simulink model "EMT_load"  (R2024a)
settings: Solver=ode1  StartTime=0.0  StopTime=simtime  FixedStep=Ts  RelTol=1e-3
values from neighbouring files (symbols this model uses):
  c0 = c0_hawk    (= 6.37282e-09)    [EMT_Phasor_parameters.m]
  c1 = c1_hawk    (= 8.76156e-09)    [EMT_Phasor_parameters.m]
  fg = 50    [EMT_Phasor_parameters.m]
  G1gen = 0.1245    [EMT_Phasor_parameters.m]
  G2gen = 0.30    (= 0.3)    [EMT_Phasor_parameters.m]
  G3gen = 0.20    (= 0.2)    [EMT_Phasor_parameters.m]
  G4sgen = 0.2078    [EMT_Phasor_parameters.m]
  G5gen = 0.20    (= 0.2)    [EMT_Phasor_parameters.m]
  G6gen = 0.2078    [EMT_Phasor_parameters.m]
  G6sgen = 0.20    (= 0.2)    [EMT_Phasor_parameters.m]
  G7gen = 0.518    [EMT_Phasor_parameters.m]
  Ihvpk = Ihv*sqrt(2)    [EMT_Phasor_parameters.m]
  l0 = l0_hawk    (= 0.00373)    [EMT_Phasor_parameters.m]
  l1 = l1_hawk    (= 0.00133)    [EMT_Phasor_parameters.m]
  L3dem = 0.10    (= 0.1)    [EMT_Phasor_parameters.m]
  L4dem = 0.30    (= 0.3)    [EMT_Phasor_parameters.m]
  L5dem = 0.35    [EMT_Phasor_parameters.m]
  L6dem = 0.15    [EMT_Phasor_parameters.m]
  L7dem = 0.10    (= 0.1)    [EMT_Phasor_parameters.m]
  Pr = Sr*PF    (= 550050000)    [EMT_Phasor_parameters.m]
  Qr = sqrt(Sr^2 - Pr^2)    [EMT_Phasor_parameters.m]
  r0 = r0_hawk    (= 0.44587)    [EMT_Phasor_parameters.m]
  r1 = r1_hawk    (= 0.12087)    [EMT_Phasor_parameters.m]
  Rtpu = Xtpu/40    (= 0.00375)    [EMT_Phasor_parameters.m]
  S1non = 400e6    (= 400000000)    [EMT_Phasor_parameters.m]
  S2non = 300e6    (= 300000000)    [EMT_Phasor_parameters.m]
  S3non = 200e6    (= 200000000)    [EMT_Phasor_parameters.m]
  S4snon = 200e6    (= 200000000)    [EMT_Phasor_parameters.m]
  S5non = 500e6    (= 500000000)    [EMT_Phasor_parameters.m]
  S6non = 400e6    (= 400000000)    [EMT_Phasor_parameters.m]
  S6snon = 200e6    (= 200000000)    [EMT_Phasor_parameters.m]
  S7non = 200e6    (= 200000000)    [EMT_Phasor_parameters.m]
  simtime = 5    [EMT_Phasor_parameters.m]
  tonvsc = 0.01    [EMT_Phasor_parameters.m]
  Ts = 150e-6    (= 0.00015)    [EMT_Phasor_parameters.m]
  Vhv = 220e3    (= 220000)    [EMT_Phasor_parameters.m]
  Vmv = 22e3    (= 22000)    [EMT_Phasor_parameters.m]
  wc1 = wsw1/10    (= 848.230016469)    [EMT_Phasor_parameters.m]
  wdc1 = wc1/10    (= 84.8230016469)    [EMT_Phasor_parameters.m]
  wpq1 = wc1/10    (= 84.8230016469)    [EMT_Phasor_parameters.m]
  wsw1 = ksw1*2*pi*fg    (= 8482.30016469)    [EMT_Phasor_parameters.m]
  Xtpu = 0.15    [EMT_Phasor_parameters.m]
undefined symbols (not defined in the file or in its folder): D11, Delta, Kf, r, theta0
libraries: simulink_extras x152, spsGroundLib x49, spsCurrentMeasurementLib x39, spsVoltageMeasurementLib x33, simulink x32, eeGeneralControl x32, slpidlib x32, powerlib x30, powerlib_meascontrol x28, spsFirstOrderFilterLib x24, eeTransforms x24, pid_lib x16
(part 13 of 16)

== system EMT_load/G5/VSC/VSC Control/Modulation/Phasor I and Phasor PQ/Inverse Park Transform (Phasor) ==
  note: Transforming from real domain to complex domain
  note: In time domain, all variables are real.
      | In phasor domain, they are complex.
      | In phasor domain, what is seen as a variation in real domain is actually an angular displacement
      | As we know that the system is balanced, d and q have the same magnitude and are shifted 90 degrees
      | Thus, having the real parts and knowing that they are shifter 90 degrees, we can recover the complex part
  dq0 : Inport
  theta : Inport  Port=2
  Complex to Magnitude-Angle : ComplexToMagnitudeAngle  Commented=on
  Constant : Constant  Commented=on  Value=exp(-1i*2*pi/3)
  Constant1 : Constant  Commented=on  Value=exp(-1i*4*pi/3)
  Constant2 : Constant  Value=0
  Demux : Demux  Outputs=2
  Demux1 : Demux  Commented=on  Outputs=3
  Exp : Math  OutputSignalType=complex
  Exp1 : Math  Commented=on  OutputSignalType=complex
  First-Order Filter1 : spsFirstOrderFilterLib/First-Order Filter  Commented=on  FilterType=Lowpass  Tc=100e-6  Ts=0  Initialize=off  Vac_Init=[0, 0, 60]  Vdc_Init=0  PlotResponse=off  FreqRange="[0,  200,  1]"
  First-Order Filter2 : spsFirstOrderFilterLib/First-Order Filter  Commented=on  FilterType=Lowpass  Tc=100e-6  Ts=0  Initialize=off  Vac_Init=[0, 0, 60]  Vdc_Init=0  PlotResponse=off  FreqRange="[0,  200,  1]"
  Gain : Gain  Commented=on  Gain=exp(-1i*2*pi/3)
  Gain1 : Gain  Gain=1/2
  Gain2 : Gain  Gain=sqrt(3)
  Gain3 : Gain  Gain=1/2
  Gain4 : Gain  Gain=sqrt(3)
  Gain5 : Gain  Gain=1i
  Gain6 : Gain  Gain=-1
  Gain7 : Gain  Commented=on  Gain=1i
  Gain8 : Gain  Commented=on  Gain=exp(-1i*4*pi/3)
  Magnitude-Angle to Complex : MagnitudeAngleToComplex  Commented=on
  Mux : Mux  Commented=on  Inputs=3
  Mux2 : Mux  Inputs=3
  Product : Product
  Product1 : Product  Commented=on
  Real-Imag to Complex : RealImagToComplex
  Real-Imag to Complex1 : RealImagToComplex
  Sum : Sum  Inputs=|++
  Sum1 : Sum  Inputs=-|-
  Sum2 : Sum  Inputs=-|+
  Terminator : Terminator  Commented=on
  Terminator1 : Terminator  Commented=on
  abc : Outport  VectorParamsAs1DForOutWhenUnconnected=off
  wires:
  ? -> Demux1/1
  Demux1/3 -> Terminator1/1
  Magnitude-Angle to Complex/1 -> Gain/1, Mux/1, Gain8/1
  Gain/1 -> Mux/2
  Complex to Magnitude-Angle/1 -> First-Order Filter1/1
  Demux1/1 -> Complex to Magnitude-Angle/1
  Mux/1 -> ?
  Gain8/1 -> Mux/3
  Demux1/2 -> Terminator/1
  Complex to Magnitude-Angle/2 -> First-Order Filter2/1
  First-Order Filter2/1 -> Magnitude-Angle to Complex/2
  First-Order Filter1/1 -> Magnitude-Angle to Complex/1
  Sum/1 -> abc/1
  Constant2/1 -> [x0]
  Exp1/1 -> Product1/2
  Gain7/1 -> Exp1/1
  Gain6/1 -> Real-Imag to Complex1/2
  [xdr] -> Gain6/1
  [xqr] -> Real-Imag to Complex/2
  [xqr] -> Real-Imag to Complex1/1
  Real-Imag to Complex1/1 -> [xq]
  [xdr] -> Real-Imag to Complex/1
  Real-Imag to Complex/1 -> [xd]
  Gain3/1 -> Mux2/3
  Gain1/1 -> Mux2/2
  Sum2/1 -> Gain3/1
  [xd] -> Gain4/1
  [xq] -> Sum2/1
  Gain4/1 -> Sum2/2
  Gain2/1 -> Sum1/2
  [xd] -> Gain2/1
  [xq] -> Sum1/1
  Sum1/1 -> Gain1/1
  [xq] -> Mux2/1
  theta/1 -> Gain5/1
  Gain5/1 -> Exp/1
  Mux2/1 -> Product/1
  Exp/1 -> Product/2
  Product/1 -> Sum/1
  [x0] -> Sum/2
  Demux/2 -> [xqr]
  Demux/1 -> [xdr]
  dq0/1 -> Demux/1

== system EMT_load/G5/VSC/VSC Control/Modulation/Phasor I and Phasor PQ/RL time constant ==
  note: Adds an RL electrical time constant to the current source
  Id* : Inport
  Iq* : Inport  Port=2
  Cartesian to Polar : simulink_extras/Transformations/Cartesian to Polar
  Corrects delay : Subsystem  Commented=on
  Polar to Cartesian : simulink_extras/Transformations/Polar to Cartesian
  Saturation : Saturate  UpperLimit=Imax  LowerLimit=0
  Sum4 : Sum  Inputs=|++
  Transfer Fcn (with initial outputs) : simulink_extras/Additional Linear/Transfer Fcn (with initial outputs)  Commented=through  N=[1]  D=[L R]  Y0=0  U0=0
  Transfer Fcn (with initial outputs)1 : simulink_extras/Additional Linear/Transfer Fcn (with initial outputs)  Commented=through  N=[1]  D=[L R]  Y0=0  U0=0
  id : Outport  VectorParamsAs1DForOutWhenUnconnected=off
  iq : Outport  Port=2  VectorParamsAs1DForOutWhenUnconnected=off
  wires:
  Corrects delay/1(dphi) -> Sum4/2
  Sum4/1 -> Polar to Cartesian/2
  Cartesian to Polar/2 -> Sum4/1
  Id*/1 -> Transfer Fcn (with initial outputs)/1
  Iq*/1 -> Transfer Fcn (with initial outputs)1/1
  Polar to Cartesian/1 -> id/1
  Polar to Cartesian/2 -> iq/1
  Transfer Fcn (with initial outputs)/1 -> Cartesian to Polar/1
  Transfer Fcn (with initial outputs)1/1 -> Cartesian to Polar/2
  Cartesian to Polar/1 -> Saturation/1
  Saturation/1 -> Polar to Cartesian/1

== system EMT_load/G5/VSC/VSC Control/Modulation/Phasor I and Phasor PQ/Subsystem ==
  note: Symmetrical components to ABC
  012 : Inport
  Gain1 : Gain  Gain=[1 a a2]  SaturateOnIntegerOverflow=on  OutDataTypeStr=Inherit: Same as input  ParamDataTypeStr=Inherit: Same as input
  Gain2 : Gain  Gain=[1 a2 a]  SaturateOnIntegerOverflow=on  OutDataTypeStr=Inherit: Same as input  ParamDataTypeStr=Inherit: Same as input
  Mux : Mux  Inputs=3
  Sum : Sum  Inputs=1  InputSameDT=on  SaturateOnIntegerOverflow=on  OutDataTypeStr=Inherit: Same as first input
  Sum1 : Sum  Inputs=1  InputSameDT=on  SaturateOnIntegerOverflow=on  OutDataTypeStr=Inherit: Same as first input
  Sum2 : Sum  Inputs=1  InputSameDT=on  SaturateOnIntegerOverflow=on  OutDataTypeStr=Inherit: Same as first input
  abc : Outport
  wires:
  Mux/1 -> abc/1
  Sum2/1 -> Mux/1
  Sum/1 -> Mux/2
  Sum1/1 -> Mux/3
  Gain1/1 -> Sum1/1
  012/1 -> Gain2/1, Sum2/1, Gain1/1
  Gain2/1 -> Sum/1

== system EMT_load/G5/VSC/VSC Control/Modulation/Phasor Quasi-EMT/Corrects delay ==
  Clock : Clock
  Gain : Gain  Gain=(2*pi*fg)
  Memory : Memory
  Sum : Sum  Inputs=|+-
  Sum2 : Sum  Inputs=|++
  Transformer connection : Constant  Commented=on  Value=pi/6
  dphi : Outport
  wires:
  Clock/1 -> Memory/1, Sum/1
  Memory/1 -> Sum/2
  Sum/1 -> Gain/1  "Ts"
  Transformer connection/1 -> Sum2/2  "Tf"
  Gain/1 -> Sum2/1
  Sum2/1 -> dphi/1

== system EMT_load/G5/VSC/VSC Control/Modulation/Phasor Quasi-EMT/Corrects delay2 ==
  Clock : Clock
  Gain : Gain  Gain=(2*pi*fg)
  Memory : Memory
  Sum : Sum  Inputs=|+-
  Sum2 : Sum  Inputs=|++
  Transformer connection : Constant  Commented=on  Value=pi/6
  dphi : Outport
  wires:
  Clock/1 -> Memory/1, Sum/1
  Memory/1 -> Sum/2
  Sum/1 -> Gain/1  "Ts"
  Transformer connection/1 -> Sum2/2  "Tf"
  Gain/1 -> Sum2/1
  Sum2/1 -> dphi/1

== system EMT_load/G5/VSC/VSC Control/Modulation/Phasor Quasi-EMT/Inverse Park Transform (Phasor) ==
  note: In time domain, all variables are real.
      | In phasor domain, they are complex.
      | In phasor domain, what is seen as a variation in real domain is actually an angular displacement
      | As we know that the system is balanced, d and q have the same magnitude and are shifted 90 degrees
      | Thus, having the real parts and knowing that they are shifter 90 degrees, we can recover the complex part
  note: Transforming from real domain to complex domain
  dq0 : Inport
  theta : Inport  Port=2
  Complex to Magnitude-Angle : ComplexToMagnitudeAngle  Commented=on
  Constant : Constant  Commented=on  Value=exp(-1i*2*pi/3)
  Constant1 : Constant  Commented=on  Value=exp(-1i*4*pi/3)
  Constant2 : Constant  Value=0
  Demux : Demux  Outputs=2
  Demux1 : Demux  Commented=on  Outputs=3
  Exp : Math  OutputSignalType=complex
  Exp1 : Math  Commented=on  OutputSignalType=complex
  First-Order Filter1 : spsFirstOrderFilterLib/First-Order Filter  Commented=on  FilterType=Lowpass  Tc=100e-6  Ts=0  Initialize=off  Vac_Init=[0, 0, 60]  Vdc_Init=0  PlotResponse=off  FreqRange="[0,  200,  1]"
  First-Order Filter2 : spsFirstOrderFilterLib/First-Order Filter  Commented=on  FilterType=Lowpass  Tc=100e-6  Ts=0  Initialize=off  Vac_Init=[0, 0, 60]  Vdc_Init=0  PlotResponse=off  FreqRange="[0,  200,  1]"
  Gain : Gain  Commented=on  Gain=exp(-1i*2*pi/3)
  Gain1 : Gain  Gain=1/2
  Gain2 : Gain  Gain=sqrt(3)
  Gain3 : Gain  Gain=1/2
  Gain4 : Gain  Gain=sqrt(3)
  Gain5 : Gain  Gain=1i
  Gain6 : Gain  Gain=-1
  Gain7 : Gain  Commented=on  Gain=1i
  Gain8 : Gain  Commented=on  Gain=exp(-1i*4*pi/3)
  Magnitude-Angle to Complex : MagnitudeAngleToComplex  Commented=on
  Mux : Mux  Commented=on  Inputs=3
  Mux2 : Mux  Inputs=3
  Product : Product
  Product1 : Product  Commented=on
  Real-Imag to Complex : RealImagToComplex
  Real-Imag to Complex1 : RealImagToComplex
  Sum : Sum  Inputs=|++
  Sum1 : Sum  Inputs=-|-
  Sum2 : Sum  Inputs=-|+
  Terminator : Terminator  Commented=on
  Terminator1 : Terminator  Commented=on
  abc : Outport  VectorParamsAs1DForOutWhenUnconnected=off
  wires:
  dq0/1 -> Demux/1
  Demux/1 -> [xdr]
  Demux/2 -> [xqr]
  [x0] -> Sum/2
  Product/1 -> Sum/1
  Exp/1 -> Product/2
  Mux2/1 -> Product/1
  Gain5/1 -> Exp/1
  theta/1 -> Gain5/1
  [xq] -> Mux2/1
  Sum1/1 -> Gain1/1
  [xq] -> Sum1/1
  [xd] -> Gain2/1
  Gain2/1 -> Sum1/2
  Gain4/1 -> Sum2/2
  [xq] -> Sum2/1
  [xd] -> Gain4/1
  Sum2/1 -> Gain3/1
  Gain1/1 -> Mux2/2
  Gain3/1 -> Mux2/3
  Real-Imag to Complex/1 -> [xd]
  [xdr] -> Real-Imag to Complex/1
  Real-Imag to Complex1/1 -> [xq]
  [xqr] -> Real-Imag to Complex1/1
  [xqr] -> Real-Imag to Complex/2
  [xdr] -> Gain6/1
  Gain6/1 -> Real-Imag to Complex1/2
  Gain7/1 -> Exp1/1
  Exp1/1 -> Product1/2
  Constant2/1 -> [x0]
  Sum/1 -> abc/1
  First-Order Filter1/1 -> Magnitude-Angle to Complex/1
  First-Order Filter2/1 -> Magnitude-Angle to Complex/2
  Complex to Magnitude-Angle/2 -> First-Order Filter2/1
  Demux1/2 -> Terminator/1
  Gain8/1 -> Mux/3
  Mux/1 -> ?
  Demux1/1 -> Complex to Magnitude-Angle/1
  Complex to Magnitude-Angle/1 -> First-Order Filter1/1
  Gain/1 -> Mux/2
  Magnitude-Angle to Complex/1 -> Gain8/1, Mux/1, Gain/1
  Demux1/3 -> Terminator1/1
  ? -> Demux1/1

== system EMT_load/G5/VSC/VSC Control/Modulation/Phasor Quasi-EMT/Subsystem ==
  note: Symmetrical components to ABC
  012 : Inport
  Gain1 : Gain  Gain=[1 a a2]  SaturateOnIntegerOverflow=on  OutDataTypeStr=Inherit: Same as input  ParamDataTypeStr=Inherit: Same as input
  Gain2 : Gain  Gain=[1 a2 a]  SaturateOnIntegerOverflow=on  OutDataTypeStr=Inherit: Same as input  ParamDataTypeStr=Inherit: Same as input
  Mux : Mux  Inputs=3
  Sum : Sum  Inputs=1  InputSameDT=on  SaturateOnIntegerOverflow=on  OutDataTypeStr=Inherit: Same as first input
  Sum1 : Sum  Inputs=1  InputSameDT=on  SaturateOnIntegerOverflow=on  OutDataTypeStr=Inherit: Same as first input
  Sum2 : Sum  Inputs=1  InputSameDT=on  SaturateOnIntegerOverflow=on  OutDataTypeStr=Inherit: Same as first input
  abc : Outport
  wires:
  Gain2/1 -> Sum/1
  012/1 -> Gain1/1, Sum2/1, Gain2/1
  Gain1/1 -> Sum1/1
  Sum1/1 -> Mux/3
  Sum/1 -> Mux/2
  Sum2/1 -> Mux/1
  Mux/1 -> abc/1

== system EMT_load/G5/VSC/VSC Control/Modulation/Phasor Quasi-EMT/V to I RL (+seq) ==
  note: d-q axis model of a 3-phase series R-L branch
  note: Using Laplace transform:
  note: Iq = (Vq1 - Vq2 - w*L*Id)/(R + s*L)
  note: Id = (Vd1 - Vd2 + w*L*Iq)/(R + s*L)
  note: V2
  note: ==========================================================================================
  note: V1
  note: Vq1 - Vq2 = [ R * Iq ] + [ L* w * Id ] + [ L * d/dt (Iq) ]
  note: where w = 2*pi*f
  note: I --->
  note: o--------| R |---| L |-------o
  note: Vd1 - Vd2 = [ R * Id ] - [ L* w * Iq ] + [ L * d/dt (Id) ]
  note: This subsystem converts the VSC output voltage in a current signal through an RL element
  Vdq1 : Inport
  Vdq2 : Inport  Port=2
  Cartesian to Polar : simulink_extras/Transformations/Cartesian to Polar
  Delay : Delay  DelayLength=1
  Demux : Demux  Outputs=2
  Mux : Mux  Inputs=2
  Polar to Cartesian : simulink_extras/Transformations/Polar to Cartesian
  R_choke1 : Gain  Gain=w*L  SaturateOnIntegerOverflow=on  OutDataTypeStr=Inherit: Same as input  ParamDataTypeStr=Inherit: Same as input
  R_choke2 : Gain  Gain=[1 -1]  SaturateOnIntegerOverflow=on  OutDataTypeStr=Inherit: Same as input  ParamDataTypeStr=Inherit: Same as input
  Saturation : Saturate  UpperLimit=Imax  LowerLimit=0
  Selector : Selector  InputPortWidth=2  IndexOptions=Index vector (dialog)  Indices=[2 1]  OutputSizes=1
  Sum : Sum  Inputs=+-+  SaturateOnIntegerOverflow=on
  Transfer Fcn (with initial outputs) : simulink_extras/Additional Linear/Transfer Fcn (with initial outputs)  N=[1]  D=[L R]  Y0=0  U0=0
  Transfer Fcn (with initial outputs)1 : simulink_extras/Additional Linear/Transfer Fcn (with initial outputs)  N=[1]  D=[L R]  Y0=0  U0=0
  idIq : Outport  VectorParamsAs1DForOutWhenUnconnected=off
  wires:
  Selector/1 -> R_choke1/1
  Vdq1/1 -> Sum/1
  R_choke1/1 -> R_choke2/1
  Sum/1 -> Demux/1
  Demux/1 -> Transfer Fcn (with initial outputs)/1
  Demux/2 -> Transfer Fcn (with initial outputs)1/1
  Polar to Cartesian/1 -> Mux/1
  Polar to Cartesian/2 -> Mux/2
  Cartesian to Polar/2 -> Polar to Cartesian/2
  Mux/1 -> Delay/1, idIq/1
  R_choke2/1 -> Sum/3
  Transfer Fcn (with initial outputs)/1 -> Cartesian to Polar/1
  Transfer Fcn (with initial outputs)1/1 -> Cartesian to Polar/2
  Vdq2/1 -> Sum/2
  Cartesian to Polar/1 -> Saturation/1
  Saturation/1 -> Polar to Cartesian/1
  Delay/1 -> Selector/1

== system EMT_load/G5/VSC/VSC Control/Modulation/Phasor Quasi-EMT/V to I RL (- seq) ==
  note: d-q axis model of a 3-phase series R-L branch
  note: Using Laplace transform:
  note: Iq = (Vq1 - Vq2 - w*L*Id)/(R + s*L)
  note: Id = (Vd1 - Vd2 + w*L*Iq)/(R + s*L)
  note: V2
  note: ==========================================================================================
  note: V1
  note: Vq1 - Vq2 = [ R * Iq ] + [ L* w * Id ] + [ L * d/dt (Iq) ]
  note: where w = 2*pi*f
  note: I --->
  note: o--------| R |---| L |-------o
  note: Vd1 - Vd2 = [ R * Id ] - [ L* w * Iq ] + [ L * d/dt (Id) ]
  note: This subsystem converts the VSC output voltage in a current signal through an RL element
  Vdq1 : Inport
  Vdq2 : Inport  Port=2
  Cartesian to Polar : simulink_extras/Transformations/Cartesian to Polar
  Delay : Delay  DelayLength=1
  Demux : Demux  Outputs=2
  Mux : Mux  Inputs=2
  Polar to Cartesian : simulink_extras/Transformations/Polar to Cartesian
  R_choke1 : Gain  Gain=w*L  SaturateOnIntegerOverflow=on  OutDataTypeStr=Inherit: Same as input  ParamDataTypeStr=Inherit: Same as input
  R_choke2 : Gain  Gain=[-1 1]  SaturateOnIntegerOverflow=on  OutDataTypeStr=Inherit: Same as input  ParamDataTypeStr=Inherit: Same as input
  Saturation : Saturate  UpperLimit=Imax  LowerLimit=0
  Selector : Selector  InputPortWidth=2  IndexOptions=Index vector (dialog)  Indices=[2 1]  OutputSizes=1
  Sum : Sum  Inputs=+-+  SaturateOnIntegerOverflow=on
  Transfer Fcn (with initial outputs) : simulink_extras/Additional Linear/Transfer Fcn (with initial outputs)  N=[1]  D=[L R]  Y0=0  U0=0
  Transfer Fcn (with initial outputs)1 : simulink_extras/Additional Linear/Transfer Fcn (with initial outputs)  N=[1]  D=[L R]  Y0=0  U0=0
  idIq : Outport  VectorParamsAs1DForOutWhenUnconnected=off
  wires:
  Selector/1 -> R_choke1/1
  Vdq1/1 -> Sum/1
  R_choke1/1 -> R_choke2/1
  Sum/1 -> Demux/1
  Demux/1 -> Transfer Fcn (with initial outputs)/1
  Demux/2 -> Transfer Fcn (with initial outputs)1/1
  Polar to Cartesian/1 -> Mux/1
  Polar to Cartesian/2 -> Mux/2
  Cartesian to Polar/2 -> Polar to Cartesian/2
  Mux/1 -> Delay/1, idIq/1
  R_choke2/1 -> Sum/3
  Transfer Fcn (with initial outputs)/1 -> Cartesian to Polar/1
  Transfer Fcn (with initial outputs)1/1 -> Cartesian to Polar/2
  Vdq2/1 -> Sum/2
  Cartesian to Polar/1 -> Saturation/1
  Saturation/1 -> Polar to Cartesian/1
  Delay/1 -> Selector/1

== system EMT_load/G6/VSC/VSC Control/Control loops/Phasor I 1st/Inner-loop ==
  note: Positive-sequence current
  note: Negative-sequence current
  iq+* : Inport
  id+* : Inport  Port=2
  iq-* : Inport  Port=3
  id-* : Inport  Port=4
  First-Order Filter{,1..3} (4 alike) : powerlib_meascontrol/Filters/First-Order Filter  FilterType=Lowpass  Tc=1/wc  Ts=0  Initialize=off  Vac_Init=[0, 0, 60]  Vdc_Init=0  PlotResponse=off  FreqRange="[0,  200,  1]"
  iq+ref : Outport
  id+ref : Outport  Port=2
  iq-ref : Outport  Port=3
  id-ref : Outport  Port=4
  wires:
  First-Order Filter3/1 -> id-ref/1
  id-*/1 -> First-Order Filter3/1
  First-Order Filter2/1 -> iq-ref/1
  iq-*/1 -> First-Order Filter2/1
  First-Order Filter1/1 -> id+ref/1
  id+*/1 -> First-Order Filter1/1
  First-Order Filter/1 -> iq+ref/1
  iq+*/1 -> First-Order Filter/1

== system EMT_load/G6/VSC/VSC Control/Control loops/Phasor I 1st/Outer-loop ==
  note: Limits the converter current
  note: Frequency droop
  note: Voltage droop
  note: Reactive power control
  note: Active power control
  note: LVRT
  Pset : Inport
  Qset : Inport  Port=2
  vqd+- : Inport  Port=3
  iqd+- : Inport  Port=4
  freq : Inport  Port=5
  Blk : Inport  Port=6
  Cartesian to Polar : simulink_extras/Transformations/Cartesian to Polar
  Compare To Constant1 : simulink/Logic and Bit Operations/Compare To Constant  relop=<  const=0  OutDataTypeStr=boolean
  Constant1 : Constant  Value=fg
  Constant10 : Constant  Value=0
  Constant11 : Constant  Value=Vlvrt0
  Constant2 : Constant  Value=Vmvpk
  Constant9 : Constant  Value=0
  Demux : Demux  Outputs=2
  Demux1 : Demux
  Demux2 : Demux
  Gain14 : Gain  Gain=1/Vmvpk
  Gain15 : Gain  Gain=Klvrt
  Gain16 : Gain  Gain=Iconvbase
  Gain5 : Gain  Gain=-1/Kfdroop*(Pconv/fg)
  Gain6 : Gain  Gain=-1/Kvdroop*(Pconv/Vmvpk)
  Mux1 : Mux  Inputs=10
  NOT : Logic  Operator=NOT  IconShape=distinctive  AllPortsSameDT=off  OutDataTypeStr=boolean
  PID Controller1 : pid_lib/PID Controller  Controller=PI  Form=Ideal  TimeDomain=Continuous-time  UseExternalTs=off  SampleTime=-1  IntegratorMethod=Forward Euler  FilterMethod=Forward Euler  ControllerParametersSource=internal  P=kp_pq  I=1/ti_pq  D=0  UseFilter=on  N=100  TunerSelectOption=Transfer Function Based (PID Tuner App)  InitialConditionSource=internal  InitialConditionForIntegrator=0  InitialConditionForFilter=0  DifferentiatorICPrevScaledInput=0  ExternalReset=none  TrackingMode=off  Kt=1  LimitOutput=off  SatLimitsSource=internal  UpperSaturationLimit=inf  LowerSaturationLimit=-inf  LinearizeAsGain=on  AntiWindupMode=none  Kb=1  POutMin=[]  POutMax=[]  IOutMin=[]  IOutMax=[]  DOutMin=[]  DOutMax=[]  NOutMin=[]  NOutMax=[]  SumOutMin=[]  SumOutMax=[]  SaturationOutMin=[]  SaturationOutMax=[]  PParamMin=[]  PParamMax=[]  IParamMin=[]  IParamMax=[]  DParamMin=[]  DParamMax=[]  NParamMin=[]  NParamMax=[]  KbParamMin=[]  KbParamMax=[]  KtParamMin=[]  KtParamMax=[]  KbOutMin=[]  KbOutMax=[]  KtOutMin=[]  KtOutMax=[]  IntegratorOutMin=[]  IntegratorOutMax=[]  FilterOutMin=[]  FilterOutMax=[]  SumI1OutMin=[]  SumI1OutMax=[]  SumI2OutMin=[]  SumI2OutMax=[]  SumI3OutMin=[]  SumI3OutMax=[]  SumI4OutMin=[]  SumI4OutMax=[]  SumDOutMin=[]  SumDOutMax=[]  DifferentiatorOutMin=[]  DifferentiatorOutMax=[]  FilterDiffOutCoefMin=[]  FilterDiffOutCoefMax=[]  ReciprocalOutMin=[]  ReciprocalOutMax=[]  SumDenOutMin=[]  SumDenOutMax=[]  SumNumOutMin=[]  SumNumOutMax=[]  DivideOutMin=[]  DivideOutMax=[]  UdiffTsProdOutMin=[]  UdiffTsProdOutMax=[]  NTsProdOutMin=[]  NTsProdOutMax=[]  UintegralTsProdOutMin=[]  UintegralTsProdOutMax=[]  UngainTsProdOutMin=[]  UngainTsProdOutMax=[]  IntegratorContinuousStateAttributes=''  IntegratorStateMustResolveToSignalObject=off  IntegratorRTWStateStorageClass=Auto  FilterContinuousStateAttributes=''  FilterStateMustResolveToSignalObject=off  FilterRTWStateStorageClass=Auto  ParallelPVariant=Passthrough  IdealPVariant=InternalParameters  IVariant=InternalParameters  DVariant=Disabled  IntegratorVariant=Continuous  SatVariant=Disabled  AWVariant=Passthrough  PCopyVariant=Disabled  TRVariant=Disabled  FdbkBlocksVariant=Forward  IdealPFdbkVariant=Disabled  SatFdbkVariant=Disabled  DerivativeFilterVariant=Disabled  NVariant=Disabled  NCopyVariant=Disabled_SignalSpec  FilterICVariant=Disabled  IntegratorICVariant=InternalICs  ExternalResetVariant=Disabled  TRSumVariant=Passthrough  SumFdbkVariant=Disabled  SumVariant=Sum_PI  TsampFilterVariant=InternalTs  TsampNgainVariant=Passthrough  TsampIntegralVariant=Passthrough  ExternalSaturationOutDataTypeStr=Inherit: Same as second input
  PID Controller6 : pid_lib/PID Controller  Controller=PI  Form=Ideal  TimeDomain=Continuous-time  UseExternalTs=off  SampleTime=-1  IntegratorMethod=Forward Euler  FilterMethod=Forward Euler  ControllerParametersSource=internal  P=kp_pq  I=1/ti_pq  D=0  UseFilter=on  N=100  TunerSelectOption=Transfer Function Based (PID Tuner App)  InitialConditionSource=internal  InitialConditionForIntegrator=0  InitialConditionForFilter=0  DifferentiatorICPrevScaledInput=0  ExternalReset=none  TrackingMode=off  Kt=1  LimitOutput=off  SatLimitsSource=internal  UpperSaturationLimit=inf  LowerSaturationLimit=-inf  LinearizeAsGain=on  AntiWindupMode=none  Kb=1  POutMin=[]  POutMax=[]  IOutMin=[]  IOutMax=[]  DOutMin=[]  DOutMax=[]  NOutMin=[]  NOutMax=[]  SumOutMin=[]  SumOutMax=[]  SaturationOutMin=[]  SaturationOutMax=[]  PParamMin=[]  PParamMax=[]  IParamMin=[]  IParamMax=[]  DParamMin=[]  DParamMax=[]  NParamMin=[]  NParamMax=[]  KbParamMin=[]  KbParamMax=[]  KtParamMin=[]  KtParamMax=[]  KbOutMin=[]  KbOutMax=[]  KtOutMin=[]  KtOutMax=[]  IntegratorOutMin=[]  IntegratorOutMax=[]  FilterOutMin=[]  FilterOutMax=[]  SumI1OutMin=[]  SumI1OutMax=[]  SumI2OutMin=[]  SumI2OutMax=[]  SumI3OutMin=[]  SumI3OutMax=[]  SumI4OutMin=[]  SumI4OutMax=[]  SumDOutMin=[]  SumDOutMax=[]  DifferentiatorOutMin=[]  DifferentiatorOutMax=[]  FilterDiffOutCoefMin=[]  FilterDiffOutCoefMax=[]  ReciprocalOutMin=[]  ReciprocalOutMax=[]  SumDenOutMin=[]  SumDenOutMax=[]  SumNumOutMin=[]  SumNumOutMax=[]  DivideOutMin=[]  DivideOutMax=[]  UdiffTsProdOutMin=[]  UdiffTsProdOutMax=[]  NTsProdOutMin=[]  NTsProdOutMax=[]  UintegralTsProdOutMin=[]  UintegralTsProdOutMax=[]  UngainTsProdOutMin=[]  UngainTsProdOutMax=[]  IntegratorContinuousStateAttributes=''  IntegratorStateMustResolveToSignalObject=off  IntegratorRTWStateStorageClass=Auto  FilterContinuousStateAttributes=''  FilterStateMustResolveToSignalObject=off  FilterRTWStateStorageClass=Auto  ParallelPVariant=Passthrough  IdealPVariant=InternalParameters  IVariant=InternalParameters  DVariant=Disabled  IntegratorVariant=Continuous  SatVariant=Disabled  AWVariant=Passthrough  PCopyVariant=Disabled  TRVariant=Disabled  FdbkBlocksVariant=Forward  IdealPFdbkVariant=Disabled  SatFdbkVariant=Disabled  DerivativeFilterVariant=Disabled  NVariant=Disabled  NCopyVariant=Disabled_SignalSpec  FilterICVariant=Disabled  IntegratorICVariant=InternalICs  ExternalResetVariant=Disabled  TRSumVariant=Passthrough  SumFdbkVariant=Disabled  SumVariant=Sum_PI  TsampFilterVariant=InternalTs  TsampNgainVariant=Passthrough  TsampIntegralVariant=Passthrough  ExternalSaturationOutDataTypeStr=Inherit: Same as second input
  Polar to Cartesian : simulink_extras/Transformations/Polar to Cartesian
  Power calculation : Subsystem
  Product3 : Product
  Saturation : Saturate  UpperLimit=Imax  LowerLimit=0
  Saturation1 : Saturate  UpperLimit=0.1*Pconv  LowerLimit=-0.1*Pconv
  Saturation2 : Saturate  UpperLimit=0.1*Pconv  LowerLimit=-0.1*Pconv
  Saturation7 : Saturate  UpperLimit=0  LowerLimit=-Qmax_lvrt
  Second-Order Filter : eeGeneralControl/Second-Order Filter  FilterType=Low-pass  fn=150  Zeta=0.9  Ts=-1  A0=0  Ph0=0  f0=0  b0=0
  Second-Order Filter1 : eeGeneralControl/Second-Order Filter  FilterType=Low-pass  fn=10  Zeta=0.9  Ts=-1  A0=50  Ph0=0  f0=0.001  b0=50
  Step : Step  Commented=on  Time=0.1  After=0.3*3711  SampleTime=0
  Step1 : Step  Commented=on  Time=0.2  After=0.2*3711  SampleTime=0
  Sum{,4,6,11} (4 alike) : Sum  Inputs=|+-
  Sum2 : Sum  Inputs=-+|
  Sum3 : Sum  Inputs=|++
  Sum5 : Sum  Inputs=|++
  Switch2 : Switch  Threshold=1  SaturateOnIntegerOverflow=off  InputSameDT=off
  Terminator : Terminator
  iq+* : Outport
  id+* : Outport  Port=2
  iq-* : Outport  Port=3
  id-* : Outport  Port=4
  m : Outport  Port=5
  wires:
  Constant10/1 -> id-*/1
  Constant9/1 -> iq-*/1
  Second-Order Filter1/1 -> Sum4/2
  [f] -> Second-Order Filter1/1
  Saturation2/1 -> Sum5/2
  Qset/1 -> Sum5/1
  Cartesian to Polar/2 -> Polar to Cartesian/2
  Polar to Cartesian/1 -> iq+*/1
  Polar to Cartesian/2 -> id+*/1
  Cartesian to Polar/1 -> Saturation/1
  Saturation/1 -> Polar to Cartesian/1
  Demux/1 -> Sum/2  "P"
  Demux/2 -> Sum2/1  "Q"
  Sum3/1 -> Sum/1  "Pref"
  Constant1/1 -> Sum4/1
  Gain5/1 -> Saturation1/1
  Sum4/1 -> Gain5/1
  Saturation1/1 -> Sum3/2
  Sum5/1 -> Sum2/2  "Qref"
  Sum6/1 -> Gain6/1
  Gain6/1 -> Saturation2/1
  [vqfilt] -> Sum6/2
  Constant2/1 -> Sum6/1
  Sum2/1 -> Product3/1
  Pset/1 -> Sum3/1
  PID Controller1/1 -> Cartesian to Polar/1
  Blk/1 -> Terminator/1
  freq/1 -> [f]
  [vqp] -> Mux1/1
  Mux1/1 -> m/1
  Product3/1 -> PID Controller6/1
  Sum/1 -> PID Controller1/1
  Second-Order Filter/1 -> [vqfilt]
  vqd+-/1 -> Demux1/1
  iqd+-/1 -> Demux2/1
  Demux1/1 -> Second-Order Filter/1, [vqp]
  Demux1/2 -> [vdp]
  Demux1/3 -> [vqn]
  Demux1/4 -> [vdn]
  Demux2/1 -> [iqp]
  Demux2/2 -> [idp]
  Demux2/3 -> [iqn]
  Demux2/4 -> [idn]
  [vqp] -> Power calculation/1(vq+)
  [iqp] -> Power calculation/3(iq+)
  Power calculation/1(PQ) -> [PQdq], Demux/1
  [idp] -> Power calculation/4(id+)
  [vdp] -> Power calculation/2(vd+)
  [vqn] -> Power calculation/5(vq-)
  [vdn] -> Power calculation/6(vd-)
  [iqn] -> Power calculation/7(iq-)
  [idn] -> Power calculation/8(id-)
  [LVRT_true] -> NOT/1
  NOT/1 -> Product3/2
  [LVRT_true] -> Switch2/2
  PID Controller6/1 -> Switch2/3
  Switch2/1 -> Cartesian to Polar/2
  Compare To Constant1/1 -> [LVRT_true]
  Gain16/1 -> Switch2/1
  Gain15/1 -> Saturation7/1
  Saturation7/1 -> Compare To Constant1/1, Gain16/1
  [vqfilt] -> Gain14/1
  Sum11/1 -> Gain15/1
  Gain14/1 -> Sum11/2
  Constant11/1 -> Sum11/1
  [vdp] -> Mux1/2
  [vqn] -> Mux1/3
  [vdn] -> Mux1/4
  [iqn] -> Mux1/7
  [idn] -> Mux1/8
  [f] -> Mux1/9
  [PQdq] -> Mux1/10
  [idp] -> Mux1/6
  [iqp] -> Mux1/5

== system EMT_load/G6/VSC/VSC Control/Control loops/Phasor I ref/Outer-loop ==
  note: LVRT
  note: Active power control
  note: Reactive power control
  note: Voltage droop
  note: Frequency droop
  note: Limits the converter current
  Pset : Inport
  Qset : Inport  Port=2
  vqd+- : Inport  Port=3
  iqd+- : Inport  Port=4
  freq : Inport  Port=5
  Blk : Inport  Port=6
  Cartesian to Polar : simulink_extras/Transformations/Cartesian to Polar
  Compare To Constant1 : simulink/Logic and Bit Operations/Compare To Constant  relop=<  const=0  OutDataTypeStr=boolean
  Constant1 : Constant  Value=fg
  Constant10 : Constant  Value=0
  Constant11 : Constant  Value=Vlvrt0
  Constant2 : Constant  Value=Vmvpk
  Constant9 : Constant  Value=0
  Demux : Demux  Outputs=2
  Demux1 : Demux
  Demux2 : Demux
  Gain : Gain  Gain=2/3 * 1/Vmvpk * wpq
  Gain1 : Gain  Gain=2/3 * 1/Vmvpk * wpq
  Gain14 : Gain  Gain=1/Vmvpk
  Gain15 : Gain  Gain=Klvrt
  Gain16 : Gain  Gain=Iconvbase
  Gain5 : Gain  Gain=-1/Kfdroop*(Pconv/fg)
  Gain6 : Gain  Gain=-1/Kvdroop*(Pconv/Vmvpk)
  Integrator : Integrator
  Integrator1 : Integrator
  Mux1 : Mux  Inputs=10
  NOT : Logic  Operator=NOT  IconShape=distinctive  AllPortsSameDT=off  OutDataTypeStr=boolean
  PID Controller1 : pid_lib/PID Controller  Commented=on  Controller=I  Form=Ideal  TimeDomain=Continuous-time  UseExternalTs=off  SampleTime=-1  IntegratorMethod=Forward Euler  FilterMethod=Forward Euler  ControllerParametersSource=internal  P=kp_pq  I=1/wpq  D=0  UseFilter=on  N=100  TunerSelectOption=Transfer Function Based (PID Tuner App)  InitialConditionSource=internal  InitialConditionForIntegrator=0  InitialConditionForFilter=0  DifferentiatorICPrevScaledInput=0  ExternalReset=none  TrackingMode=off  Kt=1  LimitOutput=off  SatLimitsSource=internal  UpperSaturationLimit=inf  LowerSaturationLimit=-inf  LinearizeAsGain=on  AntiWindupMode=none  Kb=1  POutMin=[]  POutMax=[]  IOutMin=[]  IOutMax=[]  DOutMin=[]  DOutMax=[]  NOutMin=[]  NOutMax=[]  SumOutMin=[]  SumOutMax=[]  SaturationOutMin=[]  SaturationOutMax=[]  PParamMin=[]  PParamMax=[]  IParamMin=[]  IParamMax=[]  DParamMin=[]  DParamMax=[]  NParamMin=[]  NParamMax=[]  KbParamMin=[]  KbParamMax=[]  KtParamMin=[]  KtParamMax=[]  KbOutMin=[]  KbOutMax=[]  KtOutMin=[]  KtOutMax=[]  IntegratorOutMin=[]  IntegratorOutMax=[]  FilterOutMin=[]  FilterOutMax=[]  SumI1OutMin=[]  SumI1OutMax=[]  SumI2OutMin=[]  SumI2OutMax=[]  SumI3OutMin=[]  SumI3OutMax=[]  SumI4OutMin=[]  SumI4OutMax=[]  SumDOutMin=[]  SumDOutMax=[]  DifferentiatorOutMin=[]  DifferentiatorOutMax=[]  FilterDiffOutCoefMin=[]  FilterDiffOutCoefMax=[]  ReciprocalOutMin=[]  ReciprocalOutMax=[]  SumDenOutMin=[]  SumDenOutMax=[]  SumNumOutMin=[]  SumNumOutMax=[]  DivideOutMin=[]  DivideOutMax=[]  UdiffTsProdOutMin=[]  UdiffTsProdOutMax=[]  NTsProdOutMin=[]  NTsProdOutMax=[]  UintegralTsProdOutMin=[]  UintegralTsProdOutMax=[]  UngainTsProdOutMin=[]  UngainTsProdOutMax=[]  IntegratorContinuousStateAttributes=''  IntegratorStateMustResolveToSignalObject=off  IntegratorRTWStateStorageClass=Auto  FilterContinuousStateAttributes=''  FilterStateMustResolveToSignalObject=off  FilterRTWStateStorageClass=Auto  ParallelPVariant=Disabled  IdealPVariant=Disabled  IVariant=InternalParameters  DVariant=Disabled  IntegratorVariant=Continuous  SatVariant=Disabled  AWVariant=Passthrough  PCopyVariant=Disabled  TRVariant=Disabled  FdbkBlocksVariant=Forward  IdealPFdbkVariant=Disabled  SatFdbkVariant=Disabled  DerivativeFilterVariant=Disabled  NVariant=Disabled  NCopyVariant=Disabled_SignalSpec  FilterICVariant=Disabled  IntegratorICVariant=InternalICs  ExternalResetVariant=Disabled  TRSumVariant=Passthrough  SumFdbkVariant=Disabled  SumVariant=Passthrough_I  TsampFilterVariant=InternalTs  TsampNgainVariant=Passthrough  TsampIntegralVariant=Passthrough  ExternalSaturationOutDataTypeStr=Inherit: Same as second input
  PID Controller6 : pid_lib/PID Controller  Commented=on  Controller=I  Form=Ideal  TimeDomain=Continuous-time  UseExternalTs=off  SampleTime=-1  IntegratorMethod=Forward Euler  FilterMethod=Forward Euler  ControllerParametersSource=internal  P=kp_pq  I=1/wpq  D=0  UseFilter=on  N=100  TunerSelectOption=Transfer Function Based (PID Tuner App)  InitialConditionSource=internal  InitialConditionForIntegrator=0  InitialConditionForFilter=0  DifferentiatorICPrevScaledInput=0  ExternalReset=none  TrackingMode=off  Kt=1  LimitOutput=off  SatLimitsSource=internal  UpperSaturationLimit=inf  LowerSaturationLimit=-inf  LinearizeAsGain=on  AntiWindupMode=none  Kb=1  POutMin=[]  POutMax=[]  IOutMin=[]  IOutMax=[]  DOutMin=[]  DOutMax=[]  NOutMin=[]  NOutMax=[]  SumOutMin=[]  SumOutMax=[]  SaturationOutMin=[]  SaturationOutMax=[]  PParamMin=[]  PParamMax=[]  IParamMin=[]  IParamMax=[]  DParamMin=[]  DParamMax=[]  NParamMin=[]  NParamMax=[]  KbParamMin=[]  KbParamMax=[]  KtParamMin=[]  KtParamMax=[]  KbOutMin=[]  KbOutMax=[]  KtOutMin=[]  KtOutMax=[]  IntegratorOutMin=[]  IntegratorOutMax=[]  FilterOutMin=[]  FilterOutMax=[]  SumI1OutMin=[]  SumI1OutMax=[]  SumI2OutMin=[]  SumI2OutMax=[]  SumI3OutMin=[]  SumI3OutMax=[]  SumI4OutMin=[]  SumI4OutMax=[]  SumDOutMin=[]  SumDOutMax=[]  DifferentiatorOutMin=[]  DifferentiatorOutMax=[]  FilterDiffOutCoefMin=[]  FilterDiffOutCoefMax=[]  ReciprocalOutMin=[]  ReciprocalOutMax=[]  SumDenOutMin=[]  SumDenOutMax=[]  SumNumOutMin=[]  SumNumOutMax=[]  DivideOutMin=[]  DivideOutMax=[]  UdiffTsProdOutMin=[]  UdiffTsProdOutMax=[]  NTsProdOutMin=[]  NTsProdOutMax=[]  UintegralTsProdOutMin=[]  UintegralTsProdOutMax=[]  UngainTsProdOutMin=[]  UngainTsProdOutMax=[]  IntegratorContinuousStateAttributes=''  IntegratorStateMustResolveToSignalObject=off  IntegratorRTWStateStorageClass=Auto  FilterContinuousStateAttributes=''  FilterStateMustResolveToSignalObject=off  FilterRTWStateStorageClass=Auto  ParallelPVariant=Disabled  IdealPVariant=Disabled  IVariant=InternalParameters  DVariant=Disabled  IntegratorVariant=Continuous  SatVariant=Disabled  AWVariant=Passthrough  PCopyVariant=Disabled  TRVariant=Disabled  FdbkBlocksVariant=Forward  IdealPFdbkVariant=Disabled  SatFdbkVariant=Disabled  DerivativeFilterVariant=Disabled  NVariant=Disabled  NCopyVariant=Disabled_SignalSpec  FilterICVariant=Disabled  IntegratorICVariant=InternalICs  ExternalResetVariant=Disabled  TRSumVariant=Passthrough  SumFdbkVariant=Disabled  SumVariant=Passthrough_I  TsampFilterVariant=InternalTs  TsampNgainVariant=Passthrough  TsampIntegralVariant=Passthrough  ExternalSaturationOutDataTypeStr=Inherit: Same as second input
  Polar to Cartesian : simulink_extras/Transformations/Polar to Cartesian
  Power calculation : Subsystem
  Product3 : Product
  Saturation : Saturate  UpperLimit=Imax  LowerLimit=0
  Saturation1 : Saturate  UpperLimit=0.1*Pconv  LowerLimit=-0.1*Pconv
  Saturation2 : Saturate  UpperLimit=0.1*Pconv  LowerLimit=-0.1*Pconv
  Saturation7 : Saturate  UpperLimit=0  LowerLimit=-Qmax_lvrt
  Second-Order Filter : eeGeneralControl/Second-Order Filter  FilterType=Low-pass  fn=150  Zeta=0.9  Ts=-1  A0=0  Ph0=0  f0=0  b0=0
  Second-Order Filter1 : eeGeneralControl/Second-Order Filter  FilterType=Low-pass  fn=10  Zeta=0.9  Ts=-1  A0=50  Ph0=0  f0=0.001  b0=50
  Step : Step  Commented=on  Time=0.1  After=0.3*3711  SampleTime=0
  Step1 : Step  Commented=on  Time=0.2  After=0.2*3711  SampleTime=0
  Sum{,4,6,11} (4 alike) : Sum  Inputs=|+-
  Sum2 : Sum  Inputs=-+|
  Sum3 : Sum  Inputs=|++
  Sum5 : Sum  Inputs=|++
  Switch2 : Switch  Threshold=1  SaturateOnIntegerOverflow=off  InputSameDT=off
  Terminator : Terminator
  iq+* : Outport
  id+* : Outport  Port=2
  iq-* : Outport  Port=3
  id-* : Outport  Port=4
  m : Outport  Port=5
  wires:
  Gain1/1 -> Integrator1/1
  Gain/1 -> Integrator/1
  NOT/1 -> Product3/2
  [iqp] -> Mux1/5
  [idp] -> Mux1/6
  [PQdq] -> Mux1/10
  [f] -> Mux1/9
  [idn] -> Mux1/8
  [iqn] -> Mux1/7
  [vdn] -> Mux1/4
  [vqn] -> Mux1/3
  [vdp] -> Mux1/2
  Constant11/1 -> Sum11/1
  Gain14/1 -> Sum11/2
  Sum11/1 -> Gain15/1
  [vqfilt] -> Gain14/1
  Saturation7/1 -> Gain16/1, Compare To Constant1/1
  Gain15/1 -> Saturation7/1
  Gain16/1 -> Switch2/1
  Compare To Constant1/1 -> [LVRT_true]
  Switch2/1 -> Cartesian to Polar/2
  Integrator1/1 -> Switch2/3
  [LVRT_true] -> Switch2/2
  [LVRT_true] -> NOT/1
  [idn] -> Power calculation/8(id-)
  [iqn] -> Power calculation/7(iq-)
  [vdn] -> Power calculation/6(vd-)
  [vqn] -> Power calculation/5(vq-)
  [vdp] -> Power calculation/2(vd+)
  [idp] -> Power calculation/4(id+)
  Power calculation/1(PQ) -> Demux/1, [PQdq]
  [iqp] -> Power calculation/3(iq+)
  [vqp] -> Power calculation/1(vq+)
  Demux2/4 -> [idn]
  Demux2/3 -> [iqn]
  Demux2/2 -> [idp]
  Demux2/1 -> [iqp]
  Demux1/4 -> [vdn]
  Demux1/3 -> [vqn]
  Demux1/2 -> [vdp]
  Demux1/1 -> [vqp], Second-Order Filter/1
  iqd+-/1 -> Demux2/1
  vqd+-/1 -> Demux1/1
  Second-Order Filter/1 -> [vqfilt]
  Sum/1 -> Gain/1
  Product3/1 -> Gain1/1
  Mux1/1 -> m/1
  [vqp] -> Mux1/1
  freq/1 -> [f]
  Blk/1 -> Terminator/1
  Integrator/1 -> Cartesian to Polar/1
  Pset/1 -> Sum3/1
  Sum2/1 -> Product3/1
  Constant2/1 -> Sum6/1
  [vqfilt] -> Sum6/2
  Gain6/1 -> Saturation2/1
  Sum6/1 -> Gain6/1
  Sum5/1 -> Sum2/2  "Qref"
  Saturation1/1 -> Sum3/2
  Sum4/1 -> Gain5/1
  Gain5/1 -> Saturation1/1
  Constant1/1 -> Sum4/1
  Sum3/1 -> Sum/1  "Pref"
  Demux/2 -> Sum2/1  "Q"
  Demux/1 -> Sum/2  "P"
  Saturation/1 -> Polar to Cartesian/1
  Cartesian to Polar/1 -> Saturation/1
  Polar to Cartesian/2 -> id+*/1
  Polar to Cartesian/1 -> iq+*/1
  Cartesian to Polar/2 -> Polar to Cartesian/2
  Qset/1 -> Sum5/1
  Saturation2/1 -> Sum5/2
  [f] -> Second-Order Filter1/1
  Second-Order Filter1/1 -> Sum4/2
  Constant9/1 -> iq-*/1
  Constant10/1 -> id-*/1

== system EMT_load/G6/VSC/VSC Control/Control loops/Phasor PQ 1st/Outer-loop ==
  note: Limits the converter current
  note: Frequency droop
  note: Voltage droop
  note: Reactive power control
  note: Active power control
  note: LVRT
  Pset : Inport
  Qset : Inport  Port=2
  vqd+- : Inport  Port=3
  iqd+- : Inport  Port=4
  freq : Inport  Port=5
  Blk : Inport  Port=6
  Cartesian to Polar : simulink_extras/Transformations/Cartesian to Polar
  Compare To Constant1 : simulink/Logic and Bit Operations/Compare To Constant  relop=<  const=0  OutDataTypeStr=boolean
  Constant1 : Constant  Value=fg
  Constant10 : Constant  Value=0
  Constant11 : Constant  Value=Vlvrt0
  Constant2 : Constant  Value=Vmvpk
  Constant9 : Constant  Value=0
  Demux1 : Demux
  Demux2 : Demux
  Divide1 : Product  Inputs=*/
  Divide2 : Product  Inputs=*/
  First-Order Filter : powerlib_meascontrol/Filters/First-Order Filter  FilterType=Lowpass  Tc=1/wpq  Ts=0  Initialize=off  Vac_Init=[0, 0, 60]  Vdc_Init=0  PlotResponse=off  FreqRange="[0,  200,  1]"
  First-Order Filter2 : powerlib_meascontrol/Filters/First-Order Filter  FilterType=Lowpass  Tc=1/wpq  Ts=0  Initialize=off  Vac_Init=[0, 0, 60]  Vdc_Init=0  PlotResponse=off  FreqRange="[0,  200,  1]"
  Gain : Gain  Gain=2/3
  Gain1 : Gain  Gain=2/3
  Gain14 : Gain  Gain=1/Vmvpk
  Gain15 : Gain  Gain=Klvrt
  Gain16 : Gain  Gain=Iconvbase
  Gain5 : Gain  Gain=-1/Kfdroop*(Pconv/fg)
  Gain6 : Gain  Gain=-1/Kvdroop*(Pconv/Vmvpk)
  Mux1 : Mux  Inputs=10
  Polar to Cartesian : simulink_extras/Transformations/Polar to Cartesian
  Power calculation : Subsystem
  Saturation : Saturate  UpperLimit=Imax  LowerLimit=0
  Saturation1 : Saturate  UpperLimit=0.1*Pconv  LowerLimit=-0.1*Pconv
  Saturation2 : Saturate  UpperLimit=0.1*Pconv  LowerLimit=-0.1*Pconv
  Saturation3 : Saturate  UpperLimit=inf  LowerLimit=eps
  Saturation4 : Saturate  UpperLimit=inf  LowerLimit=eps
  Saturation7 : Saturate  UpperLimit=0  LowerLimit=-Qmax_lvrt
  Second-Order Filter : eeGeneralControl/Second-Order Filter  FilterType=Low-pass  fn=150  Zeta=0.9  Ts=-1  A0=0  Ph0=0  f0=0  b0=0
  Second-Order Filter1 : eeGeneralControl/Second-Order Filter  FilterType=Low-pass  fn=10  Zeta=0.9  Ts=-1  A0=50  Ph0=0  f0=0.001  b0=50
  Step : Step  Commented=on  Time=0.1  After=0.3*3711  SampleTime=0
  Step1 : Step  Commented=on  Time=0.2  After=0.2*3711  SampleTime=0
  Sum11 : Sum  Inputs=|+-
  Sum3 : Sum  Inputs=|++
  Sum4 : Sum  Inputs=|+-
  Sum5 : Sum  Inputs=|++
  Sum6 : Sum  Inputs=|+-
  Switch2 : Switch  Threshold=1  SaturateOnIntegerOverflow=off  InputSameDT=off
  Terminator : Terminator
  iq+* : Outport
  id+* : Outport  Port=2
  iq-* : Outport  Port=3
  id-* : Outport  Port=4
  m : Outport  Port=5
  wires:
  [vqp] -> Saturation4/1
  Saturation4/1 -> Divide2/2
  Divide2/1 -> Gain1/1
  Gain1/1 -> First-Order Filter2/1
  Gain/1 -> First-Order Filter/1
  [vqp] -> Saturation3/1
  Divide1/1 -> Gain/1
  Saturation3/1 -> Divide1/2
  Constant10/1 -> id-*/1
  Constant9/1 -> iq-*/1
  Second-Order Filter1/1 -> Sum4/2
  [f] -> Second-Order Filter1/1
  Saturation2/1 -> Sum5/2
  Qset/1 -> Sum5/1
  Cartesian to Polar/2 -> Polar to Cartesian/2
  Polar to Cartesian/1 -> iq+*/1
  Polar to Cartesian/2 -> id+*/1
  Cartesian to Polar/1 -> Saturation/1
  Saturation/1 -> Polar to Cartesian/1
  Sum3/1 -> Divide1/1  "Pref"
  Constant1/1 -> Sum4/1
  Gain5/1 -> Saturation1/1
  Sum4/1 -> Gain5/1
  Saturation1/1 -> Sum3/2
  Sum5/1 -> Divide2/1  "Qref"
  Sum6/1 -> Gain6/1
  Gain6/1 -> Saturation2/1
  [vqfilt] -> Sum6/2
  Constant2/1 -> Sum6/1
  Pset/1 -> Sum3/1
  First-Order Filter/1 -> Cartesian to Polar/1
  Blk/1 -> Terminator/1
  freq/1 -> [f]
  [vqp] -> Mux1/1
  Mux1/1 -> m/1
  Second-Order Filter/1 -> [vqfilt]
  vqd+-/1 -> Demux1/1
  iqd+-/1 -> Demux2/1
  Demux1/1 -> Second-Order Filter/1, [vqp]
  Demux1/2 -> [vdp]
  Demux1/3 -> [vqn]
  Demux1/4 -> [vdn]
  Demux2/1 -> [iqp]
  Demux2/2 -> [idp]
  Demux2/3 -> [iqn]
  Demux2/4 -> [idn]
  [vqp] -> Power calculation/1(vq+)
  [iqp] -> Power calculation/3(iq+)
  Power calculation/1(PQ) -> [PQdq]
  [idp] -> Power calculation/4(id+)
  [vdp] -> Power calculation/2(vd+)
  [vqn] -> Power calculation/5(vq-)
  [vdn] -> Power calculation/6(vd-)
  [iqn] -> Power calculation/7(iq-)
  [idn] -> Power calculation/8(id-)
  [LVRT_true] -> Switch2/2
  First-Order Filter2/1 -> Switch2/3
  Switch2/1 -> Cartesian to Polar/2
  Compare To Constant1/1 -> [LVRT_true]
  Gain16/1 -> Switch2/1
  Gain15/1 -> Saturation7/1
  Saturation7/1 -> Compare To Constant1/1, Gain16/1
  [vqfilt] -> Gain14/1
  Sum11/1 -> Gain15/1
  Gain14/1 -> Sum11/2
  Constant11/1 -> Sum11/1
  [vdp] -> Mux1/2
  [vqn] -> Mux1/3
  [vdn] -> Mux1/4
  [iqn] -> Mux1/7
  [idn] -> Mux1/8
  [f] -> Mux1/9
  [PQdq] -> Mux1/10
  [idp] -> Mux1/6
  [iqp] -> Mux1/5

== system EMT_load/G6/VSC/VSC Control/Control loops/SW, EMT AVG, Phasor Quasi-EMT/Inner-loop ==
  note: Positive-sequence current control
  note: Negative-sequence current control
  iq+* : Inport
  id+* : Inport  Port=2
  iq-* : Inport  Port=3
  id-* : Inport  Port=4
  Blk : Inport  Port=5
  vqd+- : Inport  Port=6
  iqd+- : Inport  Port=7
  Demux1 : Demux
  Demux2 : Demux
  Gain{,1..3} (4 alike) : Gain  Gain=Xt
  NOT{,1..3} (4 alike) : Logic  Operator=NOT  IconShape=distinctive  AllPortsSameDT=off  OutDataTypeStr=boolean
  PID Controller{1..4} (4 alike) : slpidlib/PID Controller  Controller=PI  Form=Ideal  TimeDomain=Continuous-time  UseExternalTs=off  SampleTime=-1  IntegratorMethod=Forward Euler  FilterMethod=Forward Euler  ControllerParametersSource=internal  P=kp_c  I=1/ti_c  UseKiTs=off  D=0  UseExternalDerivativeSource=off  N=100  UseFilter=on  TunerSelectOption=Transfer Function Based (PID Tuner App)  InitialConditionSource=internal  InitialConditionForIntegrator=0  InitialConditionForFilter=0  DifferentiatorICPrevScaledInput=0  ExternalReset=level  TrackingMode=off  Kt=1  LimitOutput=off  SatLimitsSource=internal  UpperSaturationLimit=10*Vmvpk  LowerSaturationLimit=-10*Vmvpk  LinearizeAsGain=off  AntiWindupMode=none  Kb=1  LimitIntegrator=off  UpperIntegratorSaturationLimit=inf  LowerIntegratorSaturationLimit=-inf  POutMin=[]  POutMax=[]  IOutMin=[]  IOutMax=[]  DOutMin=[]  DOutMax=[]  NOutMin=[]  NOutMax=[]  SumOutMin=[]  SumOutMax=[]  SaturationOutMin=[]  SaturationOutMax=[]  PParamMin=[]  PParamMax=[]  IParamMin=[]  IParamMax=[]  DParamMin=[]  DParamMax=[]  NParamMin=[]  NParamMax=[]  KbParamMin=[]  KbParamMax=[]  KtParamMin=[]  KtParamMax=[]  KbOutMin=[]  KbOutMax=[]  KtOutMin=[]  KtOutMax=[]  IntegratorOutMin=[]  IntegratorOutMax=[]  FilterOutMin=[]  FilterOutMax=[]  SumI1OutMin=[]  SumI1OutMax=[]  SumI2OutMin=[]  SumI2OutMax=[]  SumI3OutMin=[]  SumI3OutMax=[]  SumI4OutMin=[]  SumI4OutMax=[]  SumDOutMin=[]  SumDOutMax=[]  DifferentiatorOutMin=[]  DifferentiatorOutMax=[]  FilterDiffOutCoefMin=[]  FilterDiffOutCoefMax=[]  ReciprocalOutMin=[]  ReciprocalOutMax=[]  SumDenOutMin=[]  SumDenOutMax=[]  SumNumOutMin=[]  SumNumOutMax=[]  DivideOutMin=[]  DivideOutMax=[]  UdiffTsProdOutMin=[]  UdiffTsProdOutMax=[]  NTsProdOutMin=[]  NTsProdOutMax=[]  UintegralTsProdOutMin=[]  UintegralTsProdOutMax=[]  UngainTsProdOutMin=[]  UngainTsProdOutMax=[]  ClampingZeroOutDataTypeStr=Inherit: Inherit via back propagation  ClampingZeroOutMin=[]  ClampingZeroOutMax=[]  FilterDenConstantOutDataTypeStr=Inherit: Inherit via back propagation  FilterDenConstantOutMin=[]  FilterDenConstantOutMax=[]  PCopyOutDataTypeStr=Inherit: Inherit via back propagation  PCopyOutMin=[]  PCopyOutMax=[]  NCopyOutDataTypeStr=Inherit: Inherit via back propagation  NCopyOutMin=[]  NCopyOutMax=[]  IntegratorContinuousStateAttributes=''  IntegratorStateMustResolveToSignalObject=off  IntegratorRTWStateStorageClass=Auto  FilterContinuousStateAttributes=''  FilterStateMustResolveToSignalObject=off  FilterRTWStateStorageClass=Auto  ParallelPVariant=Passthrough  IdealPVariant=InternalParameters  IVariant=InternalParameters  DVariant=Disabled  IntegratorVariant=Continuous  SatVariant=Disabled  AWVariant=Passthrough  PCopyVariant=Disabled  TRVariant=Disabled  FdbkBlocksVariant=Forward  IdealPFdbkVariant=Disabled  SatFdbkVariant=Disabled  DerivativeFilterVariant=Disabled  NVariant=Disabled  NCopyVariant=Disabled_SignalSpec  FilterICVariant=Disabled  IntegratorICVariant=InternalICs  ExternalResetVariant=ExternalReset  TRSumVariant=Passthrough  SumFdbkVariant=Disabled  SumVariant=Sum_PI  TsampFilterVariant=InternalTs  TsampNgainVariant=Passthrough  TsampIntegralVariant=Disabled_SignalSpec  ExternalSaturationOutDataTypeStr=Inherit: Same as second input  DerivativeSourceVariant=Disabled
  Product{,1..3} (4 alike) : Product
  Sum : Sum  Inputs=|+-
  Sum1 : Sum  Inputs=+-+
  Sum2 : Sum  Inputs=+--
  Sum3 : Sum  Inputs=-+|
  Sum4 : Sum  Inputs=|+-
  Sum5 : Sum  Inputs=--+
  Sum6 : Sum  Inputs=+-+
  Sum7 : Sum  Inputs=-+|
  vq+* : Outport
  vd+* : Outport  Port=2
  vq-* : Outport  Port=3
  vd-* : Outport  Port=4
  wires:
  [vdp] -> Sum1/3
  iq+*/1 -> Sum/1
  [iqp] -> Gain1/1, Sum/2
  [idp] -> Gain/1, Sum3/1
  PID Controller3/1 -> Sum1/2
  Gain1/1 -> Sum1/1
  PID Controller2/1 -> Sum2/2
  Gain/1 -> Sum2/3
  id+*/1 -> Sum3/2
  Blk/1 -> [blk]
  [blk] -> NOT/1, PID Controller2/2
  Product/1 -> PID Controller2/1
  Sum/1 -> Product/1
  NOT/1 -> Product/2
  [blk] -> PID Controller3/2, NOT1/1
  NOT1/1 -> Product1/2
  Sum3/1 -> Product1/1
  Product1/1 -> PID Controller3/1
  Sum1/1 -> vd+*/1
  Sum2/1 -> vq+*/1
  [vqp] -> Sum2/1
  Demux2/2 -> [idp]
  iqd+-/1 -> Demux2/1
  Demux2/4 -> [idn]
  Demux1/3 -> [vqn]
  Demux1/2 -> [vdp]
  Demux1/4 -> [vdn]
  Demux1/1 -> [vqp]
  Demux2/3 -> [iqn]
  Demux2/1 -> [iqp]
  vqd+-/1 -> Demux1/1
  iq-*/1 -> Sum4/1
  [blk] -> PID Controller4/2, NOT3/1
  Sum5/1 -> vd-*/1
  NOT2/1 -> Product2/2
  Sum7/1 -> Product3/1
  id-*/1 -> Sum7/2
  PID Controller4/1 -> Sum5/2
  NOT3/1 -> Product3/2
  Product3/1 -> PID Controller4/1
  PID Controller1/1 -> Sum6/2
  Product2/1 -> PID Controller1/1
  Sum4/1 -> Product2/1
  Gain3/1 -> Sum5/1
  Sum6/1 -> vq-*/1
  [blk] -> NOT2/1, PID Controller1/2
  Gain2/1 -> Sum6/3
  [idn] -> Gain2/1, Sum7/1
  [iqn] -> Sum4/2, Gain3/1
  [vqn] -> Sum6/1
  [vdn] -> Sum5/3
